simulink model "parallel_delay_compensation_6phase"  (R2022a)
settings: Solver=FixedStepDiscrete  StartTime=0.0  StopTime=10.0  RelTol=1e-3
undefined symbols (not defined in the file or in its folder): f_c, L_d, L_q, L_x, L_y, p, psi_pm, R_ph
libraries: hdlsllib x2
settings Model: DataTypeOverride=Off  Creator=Andre Merx  LastModifiedBy=Andre Merx
settings SolverCC: AlgebraicLoopSolver=TrustRegion
settings DataIOCC: LimitDataPoints=on  SaveOutput=off  SaveTime=off
settings OptimizationCC: BlockReduction=off  ConditionallyExecuteInputs=off  DefaultParameterBehavior=Inlined  LifeSpan=inf
settings DebuggingCC: AlgebraicLoopMsg=error  SingleTaskRateTransMsg=error  UnconnectedInputMsg=warning  UnconnectedOutputMsg=warning  UnconnectedLineMsg=warning  AllowSymbolicDim=off  StrictBusMsg=ErrorOnBusTreatedAsVector  SFUnexpectedBacktrackingDiag=warning  SFNoUnconditionalDefaultTransitionDiag=warning  SFExecutionAtInitializationDiag=none  SFMachineParentedDataDiag=warning  ArithmeticOperatorsInVariantConditions=warning
settings HardwareCC: ProdBitPerPointer=32  ProdBitPerSizeT=32  ProdBitPerPtrDiffT=32  ProdLargestAtomicFloat=None  ProdIntDivRoundTo=Undefined  ProdEndianess=Unspecified  ProdWordSize=32  ProdHWDeviceType=ASIC/FPGA->ASIC/FPGA  ProdEqTarget=off
settings SFSimCC: SimUseLocalCustomCode=off  CustomCodeUndefinedFunction=UseInterfaceOnly
settings RTWCC: RTWUseLocalCustomCode=off
settings CodeAppCC: StateflowObjectComments=on
settings GRTTargetCC: TargetLangStandard=C89/C90 (ANSI)
settings ConfigComp: CovScope=ReferencedModels  CovMetricSettings=dw  CovSaveCumulativeToWorkspaceVar=on  CovSaveSingleToWorkspaceVar=on  CovExternalEMLEnable=off  CovSFcnEnable=off

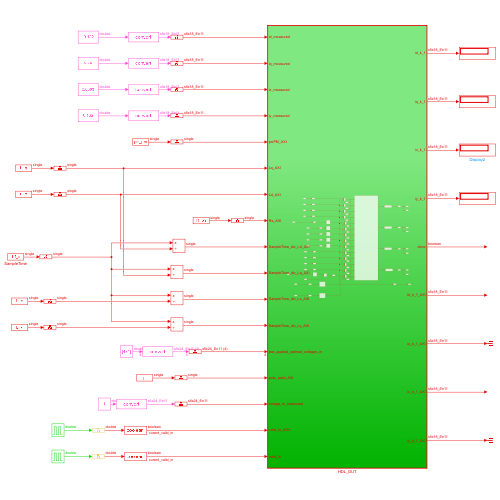
[thumbnail: Simulink's stored preview of the top-level diagram]
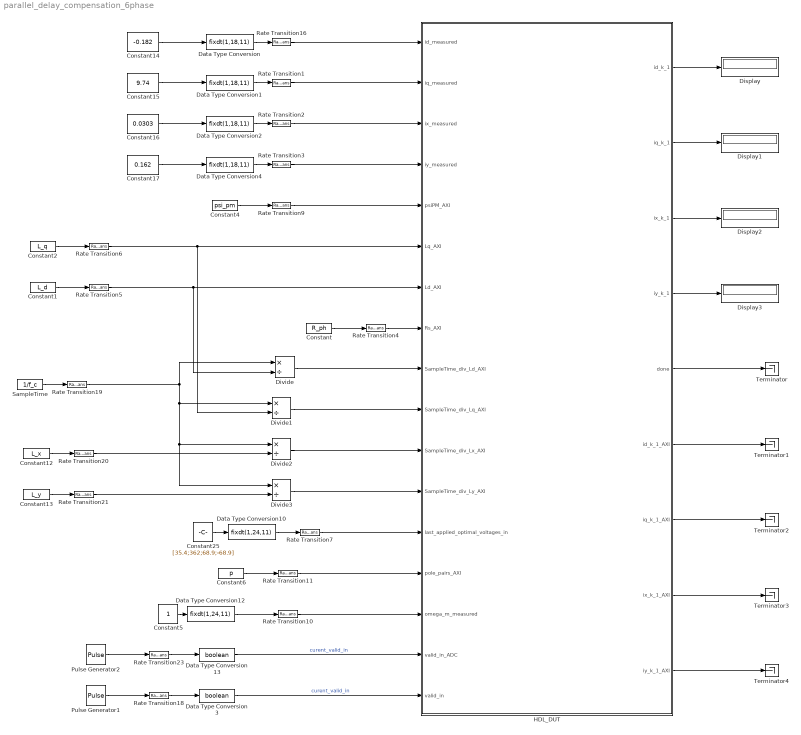
== system parallel_delay_compensation_6phase ==
  Constant : Constant  Value=R_ph  OutDataTypeStr=single  SampleTime=-1
  Constant1 : Constant  Value=L_d  OutDataTypeStr=single  SampleTime=-1
  Constant12 : Constant  Value=L_x  OutDataTypeStr=single  SampleTime=-1
  Constant13 : Constant  Value=L_y  OutDataTypeStr=single  SampleTime=-1
  Constant14 : Constant  Value=-0.182
  Constant15 : Constant  Value=9.74
  Constant16 : Constant  Value=0.0303
  Constant17 : Constant  Value=0.162
  Constant2 : Constant  Value=L_q  OutDataTypeStr=single  SampleTime=-1
  Constant25 : Constant  Value=[35.4;362;68.9;-68.9]
  Constant4 : Constant  Value=psi_pm  OutDataTypeStr=single  SampleTime=-1
  Constant5 : Constant
  Constant6 : Constant  Value=p  OutDataTypeStr=single  SampleTime=-1
  Data Type Conversion{,1..2,4} (4 alike) : DataTypeConversion  OutDataTypeStr=fixdt(1,18,11)  SaturateOnIntegerOverflow=off  RndMeth=Floor
  Data Type Conversion10 : DataTypeConversion  OutDataTypeStr=fixdt(1,24,11)  SaturateOnIntegerOverflow=off  RndMeth=Floor
  Data Type Conversion12 : DataTypeConversion  OutDataTypeStr=fixdt(1,24,11)  SaturateOnIntegerOverflow=off  RndMeth=Floor
  Data Type Conversion13 : DataTypeConversion  OutDataTypeStr=boolean  SaturateOnIntegerOverflow=off  RndMeth=Floor
  Data Type Conversion3 : DataTypeConversion  OutDataTypeStr=boolean  SaturateOnIntegerOverflow=off  RndMeth=Floor
  Display{,1..3} (4 alike) : Display
  Divide{,1..3} (4 alike) : Product  Inputs=*/  RndMeth=Zero  SaturateOnIntegerOverflow=on
  HDL_DUT : Subsystem  TreatAsAtomicUnit=on
  Pulse Generator1 : DiscretePulseGenerator  PulseType=Time based  Period=1/f_c
  Pulse Generator2 : DiscretePulseGenerator  PulseType=Time based  Period=1/f_c
  Rate Transition{1..7,9..11,16,18..21,23} (16 alike) : RateTransition  OutPortSampleTime=Rt
  SampleTime : Constant  Value=1/f_c  OutDataTypeStr=single  SampleTime=-1
  Terminator{,1..4} (5 alike) : Terminator
  wires:
  Constant25/1 -> Data Type Conversion10/1
  Divide/1 -> HDL_DUT/9(SampleTime_div_Ld_AXI)
  SampleTime/1 -> Rate Transition19/1
  Divide2/1 -> HDL_DUT/11(SampleTime_div_Lx_AXI)
  Rate Transition21/1 -> Divide3/2
  Rate Transition18/1 -> Data Type Conversion3/1
  Divide3/1 -> HDL_DUT/12(SampleTime_div_Ly_AXI)
  Rate Transition20/1 -> Divide2/2
  Rate Transition11/1 -> HDL_DUT/14(pole_pairs_AXI)
  Divide1/1 -> HDL_DUT/10(SampleTime_div_Lq_AXI)
  Rate Transition19/1 -> Divide/1, Divide1/1, Divide3/1, Divide2/1
  Constant13/1 -> Rate Transition21/1
  Constant12/1 -> Rate Transition20/1
  Pulse Generator1/1 -> Rate Transition18/1
  Data Type Conversion3/1 -> HDL_DUT/17(valid_in)  "curent_valid_in"
  Constant2/1 -> Rate Transition6/1
  Constant1/1 -> Rate Transition5/1
  Rate Transition6/1 -> HDL_DUT/6(Lq_AXI), Divide1/2
  Constant/1 -> Rate Transition4/1
  Data Type Conversion12/1 -> Rate Transition10/1
  Constant5/1 -> Data Type Conversion12/1
  Rate Transition9/1 -> HDL_DUT/5(psiPM_AXI)
  Rate Transition10/1 -> HDL_DUT/15(omega_m_measured)
  Rate Transition2/1 -> HDL_DUT/3(ix_measured)
  Rate Transition3/1 -> HDL_DUT/4(iy_measured)
  Constant14/1 -> Data Type Conversion/1
  Data Type Conversion1/1 -> Rate Transition1/1
  Data Type Conversion2/1 -> Rate Transition2/1
  Constant4/1 -> Rate Transition9/1
  Data Type Conversion/1 -> Rate Transition16/1
  Constant16/1 -> Data Type Conversion2/1
  Constant6/1 -> Rate Transition11/1
  Rate Transition5/1 -> HDL_DUT/7(Ld_AXI), Divide/2
  Rate Transition4/1 -> HDL_DUT/8(Rs_AXI)
  Data Type Conversion4/1 -> Rate Transition3/1
  Rate Transition1/1 -> HDL_DUT/2(iq_measured)
  Constant15/1 -> Data Type Conversion1/1
  Rate Transition16/1 -> HDL_DUT/1(id_measured)
  Constant17/1 -> Data Type Conversion4/1
  HDL_DUT/1(id_k_1) -> Display/1
  HDL_DUT/2(iq_k_1) -> Display1/1
  HDL_DUT/3(ix_k_1) -> Display2/1
  HDL_DUT/4(iy_k_1) -> Display3/1
  HDL_DUT/5(done) -> Terminator/1
  Data Type Conversion10/1 -> Rate Transition7/1
  HDL_DUT/6(id_k_1_AXI) -> Terminator1/1
  HDL_DUT/7(iq_k_1_AXI) -> Terminator2/1
  HDL_DUT/8(ix_k_1_AXI) -> Terminator3/1
  HDL_DUT/9(iy_k_1_AXI) -> Terminator4/1
  Pulse Generator2/1 -> Rate Transition23/1
  Rate Transition23/1 -> Data Type Conversion13/1
  Data Type Conversion13/1 -> HDL_DUT/16(valid_in_ADC)  "curent_valid_in"
  Rate Transition7/1 -> HDL_DUT/13(last_applied_optimal_voltages_in)

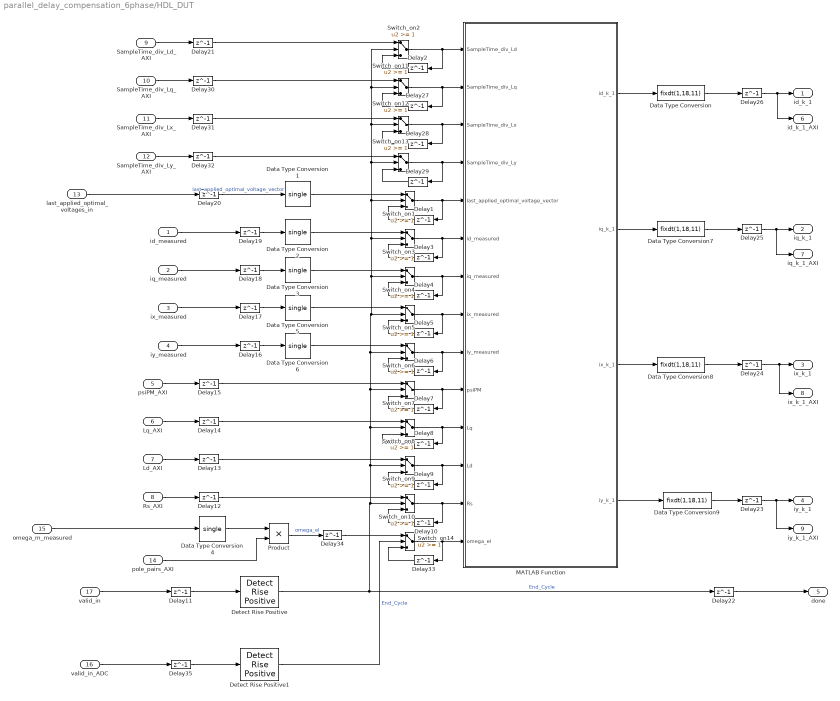
== system parallel_delay_compensation_6phase/HDL_DUT ==
  id_measured : Inport
  iq_measured : Inport  Port=2
  ix_measured : Inport  Port=3
  iy_measured : Inport  Port=4
  psiPM_AXI : Inport  Port=5
  Lq_AXI : Inport  Port=6
  Ld_AXI : Inport  Port=7
  Rs_AXI : Inport  Port=8
  SampleTime_div_Ld_AXI : Inport  Port=9
  SampleTime_div_Lq_AXI : Inport  Port=10
  SampleTime_div_Lx_AXI : Inport  Port=11
  SampleTime_div_Ly_AXI : Inport  Port=12
  last_applied_optimal_voltages_in : Inport  Port=13
  pole_pairs_AXI : Inport  Port=14
  omega_m_measured : Inport  Port=15
  valid_in_ADC : Inport  Port=16
  valid_in : Inport  Port=17
  Data Type Conversion{,7..9} (4 alike) : DataTypeConversion  OutDataTypeStr=fixdt(1,18,11)  SaturateOnIntegerOverflow=off  RndMeth=Floor
  Data Type Conversion{1..6} (6 alike) : DataTypeConversion  OutDataTypeStr=single  RndMeth=Nearest  SaturateOnIntegerOverflow=off
  Delay{1..35} (35 alike) : Delay  DelayLength=1
  Detect Rise Positive : hdlsllib/Logic and Bit Operations/Detect Rise Positive  vinit=0  OutDataTypeStr=boolean
      settings: SourceProductBaseCode=SL
  Detect Rise Positive1 : hdlsllib/Logic and Bit Operations/Detect Rise Positive  vinit=0  OutDataTypeStr=boolean
      settings: SourceProductBaseCode=SL
  MATLAB Function : MATLAB Function  TreatAsAtomicUnit=on
  Product : Product  Inputs=**
  Switch_on{1..14} (14 alike) : Switch  Threshold=1  OutDataTypeStr=single  RndMeth=Simplest  SaturateOnIntegerOverflow=off  InputSameDT=off
  id_k_1 : Outport
  iq_k_1 : Outport  Port=2
  ix_k_1 : Outport  Port=3
  iy_k_1 : Outport  Port=4
  done : Outport  Port=5
  id_k_1_AXI : Outport  Port=6
  iq_k_1_AXI : Outport  Port=7
  ix_k_1_AXI : Outport  Port=8
  iy_k_1_AXI : Outport  Port=9
  wires:
  Switch_on14/1 -> MATLAB Function/14(omega_el), Delay33/1
  Delay33/1 -> Switch_on14/3
  pole_pairs_AXI/1 -> Product/2
  Data Type Conversion4/1 -> Product/1
  Delay9/1 -> Switch_on9/3
  Delay16/1 -> Data Type Conversion6/1
  Switch_on9/1 -> Delay9/1, MATLAB Function/12(Ld)
  Delay32/1 -> Switch_on13/1
  MATLAB Function/2(iq_k_1) -> Data Type Conversion7/1
  Lq_AXI/1 -> Delay14/1
  Delay31/1 -> Switch_on12/1
  Switch_on12/1 -> MATLAB Function/3(SampleTime_div_Lx), Delay28/1
  Delay30/1 -> Switch_on11/1
  Delay29/1 -> Switch_on13/3
  SampleTime_div_Lx_AXI/1 -> Delay31/1
  Delay26/1 -> id_k_1_AXI/1, id_k_1/1
  Detect Rise Positive/1 -> Switch_on13/2, Switch_on12/2, Switch_on2/2, Switch_on11/2, Switch_on1/2, Switch_on3/2, Switch_on4/2, Switch_on5/2, Switch_on6/2, Switch_on7/2, Switch_on8/2, Switch_on9/2, Switch_on10/2, Delay22/1  "End_Cycle"
  Product/1 -> Delay34/1  "omega_el"
  Delay11/1 -> Detect Rise Positive/1
  Delay2/1 -> Switch_on2/3
  SampleTime_div_Lq_AXI/1 -> Delay30/1
  Switch_on5/1 -> Delay5/1, MATLAB Function/8(ix_measured)
  Delay12/1 -> Switch_on10/1
  Rs_AXI/1 -> Delay12/1
  Delay1/1 -> Switch_on1/3
  MATLAB Function/3(ix_k_1) -> Data Type Conversion8/1
  Delay27/1 -> Switch_on11/3
  Delay21/1 -> Switch_on2/1
  Delay23/1 -> iy_k_1_AXI/1, iy_k_1/1
  MATLAB Function/1(id_k_1) -> Data Type Conversion/1
  Delay24/1 -> ix_k_1_AXI/1, ix_k_1/1
  Delay20/1 -> Data Type Conversion1/1  "last_applied_optimal_voltage_vector"
  Delay17/1 -> Data Type Conversion5/1
  Switch_on1/1 -> Delay1/1, MATLAB Function/5(last_applied_optimal_voltage_vector)
  Delay19/1 -> Data Type Conversion2/1
  Delay8/1 -> Switch_on8/3
  Delay10/1 -> Switch_on10/3
  valid_in/1 -> Delay11/1
  Delay18/1 -> Data Type Conversion3/1
  Switch_on6/1 -> Delay6/1, MATLAB Function/9(iy_measured)
  MATLAB Function/4(iy_k_1) -> Data Type Conversion9/1
  psiPM_AXI/1 -> Delay15/1
  Delay25/1 -> iq_k_1_AXI/1, iq_k_1/1
  Switch_on13/1 -> MATLAB Function/4(SampleTime_div_Ly), Delay29/1
  Switch_on4/1 -> Delay4/1, MATLAB Function/7(iq_measured)
  Delay15/1 -> Switch_on7/1
  SampleTime_div_Ly_AXI/1 -> Delay32/1
  Switch_on10/1 -> Delay10/1, MATLAB Function/13(Rs)
  Switch_on7/1 -> Delay7/1, MATLAB Function/10(psiPM)
  Delay7/1 -> Switch_on7/3
  Delay28/1 -> Switch_on12/3
  Switch_on8/1 -> Delay8/1, MATLAB Function/11(Lq)
  Ld_AXI/1 -> Delay13/1
  Delay6/1 -> Switch_on6/3
  Delay4/1 -> Switch_on4/3
  Switch_on11/1 -> Delay27/1, MATLAB Function/2(SampleTime_div_Lq)
  Delay3/1 -> Switch_on3/3
  Delay14/1 -> Switch_on8/1
  Switch_on2/1 -> Delay2/1, MATLAB Function/1(SampleTime_div_Ld)
  Delay22/1 -> done/1
  Switch_on3/1 -> Delay3/1, MATLAB Function/6(id_measured)
  Delay13/1 -> Switch_on9/1
  Delay5/1 -> Switch_on5/3
  SampleTime_div_Ld_AXI/1 -> Delay21/1
  Data Type Conversion1/1 -> Switch_on1/1
  Data Type Conversion2/1 -> Switch_on3/1
  Data Type Conversion3/1 -> Switch_on4/1
  Data Type Conversion5/1 -> Switch_on5/1
  last_applied_optimal_voltages_in/1 -> Delay20/1
  id_measured/1 -> Delay19/1
  iq_measured/1 -> Delay18/1
  ix_measured/1 -> Delay17/1
  Data Type Conversion6/1 -> Switch_on6/1
  iy_measured/1 -> Delay16/1
  omega_m_measured/1 -> Data Type Conversion4/1
  Data Type Conversion/1 -> Delay26/1
  Data Type Conversion7/1 -> Delay25/1
  Data Type Conversion8/1 -> Delay24/1
  Data Type Conversion9/1 -> Delay23/1
  Delay34/1 -> Switch_on14/1
  Delay35/1 -> Detect Rise Positive1/1
  Detect Rise Positive1/1 -> Switch_on14/2  "End_Cycle"
  valid_in_ADC/1 -> Delay35/1

== matlab function parallel_delay_compensation_6phase/HDL_DUT/MATLAB Function ==
  data: SampleTime_div_Ld input; SampleTime_div_Lq input; SampleTime_div_Lx input; SampleTime_div_Ly input; id_k_1 output; last_applied_optimal_voltage_vector input; id_measured input; iq_measured input; ix_measured input; iy_measured input; psiPM input; Lq input; Ld input; Rs input; iq_k_1 output; ix_k_1 output; iy_k_1 output; omega_el input
function [id_k_1, iq_k_1, ix_k_1, iy_k_1] = fcn(SampleTime_div_Ld, SampleTime_div_Lq, SampleTime_div_Lx, SampleTime_div_Ly, last_applied_optimal_voltage_vector, id_measured, iq_measured, ix_measured, iy_measured, psiPM, Lq, Ld, Rs, omega_el)
  
    % Delay compensation with a modell of a 6-Phase PMSM
    id_k_1 = single(SampleTime_div_Ld*(last_applied_optimal_voltage_vector(1)-id_measured*Rs+omega_el*Lq*iq_measured)+id_measured);
    iq_k_1 = single(SampleTime_div_Lq*(last_applied_optimal_voltage_vector(2)-iq_measured*Rs-omega_el*(psiPM+id_measured*Ld))+iq_measured);
    ix_k_1 = single(SampleTime_div_Lx*(last_applied_optimal_voltage_vector(3)-ix_measured*Rs)+ix_measured);
    iy_k_1 = single(SampleTime_div_Ly*(last_applied_optimal_voltage_vector(4)-iy_measured*Rs)+iy_measured);

end
